simulink model "chairforceone"  (R2024a)
settings: Solver=FixedStepAuto  StartTime=0.0  StopTime=inf  RelTol=1e-3
libraries: robotlib x5
settings Model: Creator=carlosortiz  LastModifiedBy=suryachand
settings OptimizationCC: EnhancedBackFolding=on  PassReuseOutputArgsAs=Individual arguments  MaxStackSize=64  OptimizeBlockOrder=speed  DifferentSizesBufferReuse=on  OptimizationCustomize=off  EfficientTunableParamExpr=on
settings DebuggingCC: ParameterTunabilityLossMsg=error
settings HardwareCC: ProdBitPerPointer=32  ProdBitPerSizeT=32  ProdBitPerPtrDiffT=32  ProdLargestAtomicFloat=None  ProdIntDivRoundTo=Undefined  ProdEndianess=Unspecified  ProdWordSize=32  ProdHWDeviceType=Generic->Unspecified (assume 32-bit Generic)  UseEmbeddedCoderFeatures=off
settings SFSimCC: MATLABDynamicMemAlloc=off
settings RTWCC: Description=Embedded Coder  SystemTargetFile=ert.tlc  HardwareBoard=Robot Operating System (ROS)  TLCOptions="-aInlineSetEventsForThisBaseRateFcn=TLC_FALSE -aSuppressMultiTaskScheduler=TLC_FALSE  -aRateBasedStepFcn=0"  TemplateMakefile=ert_default_tmf  Toolchain=Catkin  TargetLang=C++
settings CodeAppCC: ForceParamTrailComments=on  IgnoreCustomStorageClasses=off  OperatorAnnotations=on  SimulinkDataObjDesc=on  SFDataObjDesc=on  InsertBlockDesc=on
settings ERTTargetCC: SupportNonInlinedSFcns=on

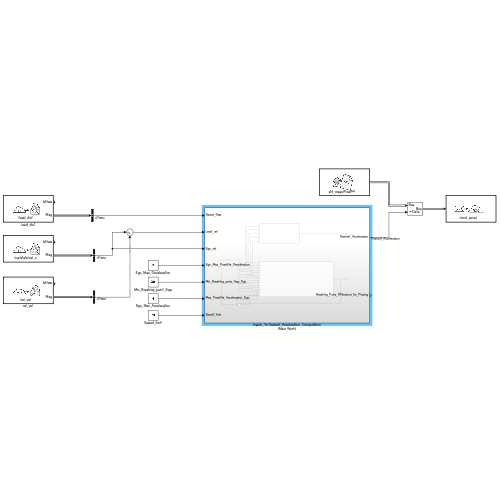
[thumbnail: Simulink's stored preview of the top-level diagram]
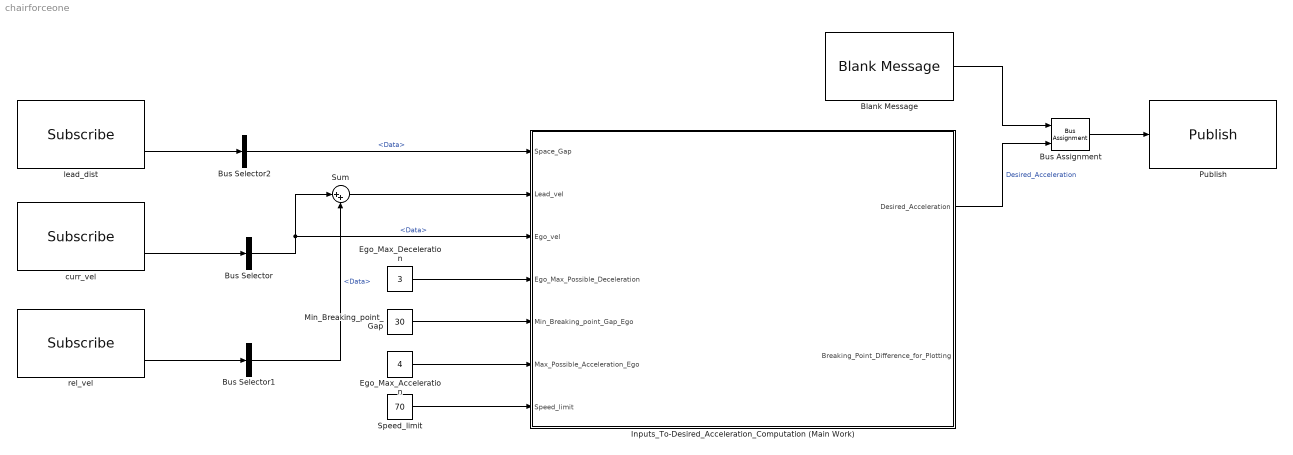
== system chairforceone ==
  Blank Message : robotlib/Blank Message  messageClass=Message  entityType=std_msgs/Float64  messageType=std_msgs/Float64  SampleTime=inf  legacyBusStruct=off
  Bus Assignment : BusAssignment  AssignedSignals=Data
  Bus Selector : BusSelector  OutputSignals=Data
  Bus Selector1 : BusSelector  OutputSignals=Data
  Bus Selector2 : BusSelector  OutputSignals=Data
  Ego_Max_Acceleration : Constant  Value=4
  Ego_Max_Deceleration : Constant  Value=3
  Inputs_To-Desired_Acceleration_Computation (Main Work) : Subsystem
  Min_Breaking_point_Gap : Constant  Value=30
  Publish : robotlib/Publish  topicSource=Specify your own  topic=/cmd_accel  messageType=std_msgs/Float64  legacyBusStruct=off  messageQueueLength=1
  Speed_limit : Constant  Value=70
  Sum : Sum  Inputs=|++
  curr_vel : robotlib/Subscribe  topicSource=Specify your own  topic=/car/state/vel_x  messageType=std_msgs/Float64  SampleTime=-1  legacyBusStruct=off  messageQueueLength=1
  lead_dist : robotlib/Subscribe  topicSource=Specify your own  topic=/lead_dist  messageType=std_msgs/Float64  SampleTime=-1  legacyBusStruct=off  messageQueueLength=1
  rel_vel : robotlib/Subscribe  topicSource=Specify your own  topic=/rel_vel  messageType=std_msgs/Float64  SampleTime=-1  legacyBusStruct=off  messageQueueLength=1
  wires:
  curr_vel/2 -> Bus Selector/1
  rel_vel/2 -> Bus Selector1/1
  lead_dist/2 -> Bus Selector2/1
  Bus Selector2/1 -> Inputs_To-Desired_Acceleration_Computation (Main Work)/1(Space_Gap)  "<Data>"
  Bus Selector/1 -> Sum/1, Inputs_To-Desired_Acceleration_Computation (Main Work)/3(Ego_vel)  "<Data>"
  Sum/1 -> Inputs_To-Desired_Acceleration_Computation (Main Work)/2(Lead_vel)
  Bus Selector1/1 -> Sum/2  "<Data>"
  Blank Message/1 -> Bus Assignment/1
  Inputs_To-Desired_Acceleration_Computation (Main Work)/1(Desired_Acceleration) -> Bus Assignment/2  "Desired_Acceleration"
  Bus Assignment/1 -> Publish/1
  Ego_Max_Deceleration/1 -> Inputs_To-Desired_Acceleration_Computation (Main Work)/4(Ego_Max_Possible_Deceleration)
  Min_Breaking_point_Gap/1 -> Inputs_To-Desired_Acceleration_Computation (Main Work)/5(Min_Breaking_point_Gap_Ego)
  Ego_Max_Acceleration/1 -> Inputs_To-Desired_Acceleration_Computation (Main Work)/6(Max_Possible_Acceleration_Ego)
  Speed_limit/1 -> Inputs_To-Desired_Acceleration_Computation (Main Work)/7(Speed_limit)

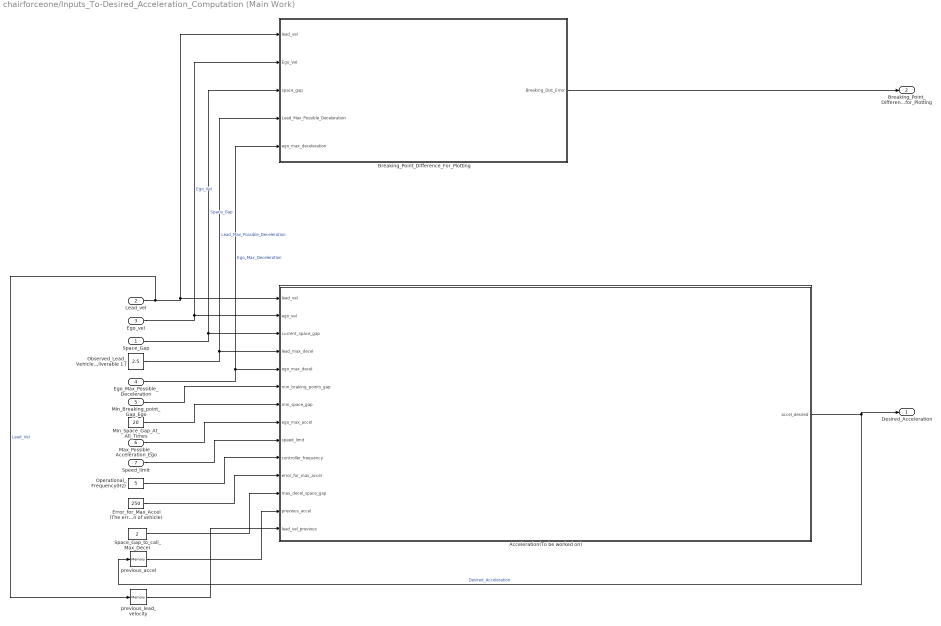
== system chairforceone/Inputs_To-Desired_Acceleration_Computation (Main Work) ==
  Space_Gap : Inport
  Lead_vel : Inport  Port=2
  Ego_vel : Inport  Port=3
  Ego_Max_Possible_Deceleration : Inport  Port=4
  Min_Breaking_point_Gap_Ego : Inport  Port=5
  Max_Possible_Acceleration_Ego : Inport  Port=6
  Speed_limit : Inport  Port=7
  Acceleration(To be worked on) : MATLAB Function  TreatAsAtomicUnit=on
  Breaking_Point_Difference_For_Plotting : Subsystem
  Error_for_Max_Accel (The error distance in breaking points which is threshold for using max acceleration of vehicle) : Constant  Value=250
  Min_Space_Gap_At_All_Times : Constant  Value=20
  Observed_Lead_Vehicle_Max_Deceleration (For now keeping one fixed value to all vehicles for scope of deliverable 1 ) : Constant  Value=2.5
  Operational_Frequency(Hz) : Constant  Value=5
  Space_Gap_to_call_Max_Decel : Constant  Value=2
  previous_accel : Memory
  previous_lead_velocity : Memory
  Desired_Acceleration : Outport
  Breaking_Point_Difference_for_Plotting : Outport  Port=2
  wires:
  Acceleration(To be worked on)/1(accel_desired) -> Desired_Acceleration/1, previous_accel/1  "Desired_Acceleration"
  Min_Breaking_point_Gap_Ego/1 -> Acceleration(To be worked on)/6(min_braking_points_gap)
  Max_Possible_Acceleration_Ego/1 -> Acceleration(To be worked on)/8(ego_max_accel)
  Speed_limit/1 -> Acceleration(To be worked on)/9(speed_limit)
  Min_Space_Gap_At_All_Times/1 -> Acceleration(To be worked on)/7(min_space_gap)
  Operational_Frequency(Hz)/1 -> Acceleration(To be worked on)/10(controller_frequency)
  Error_for_Max_Accel (The error distance in breaking points which is threshold for using max acceleration of vehicle)/1 -> Acceleration(To be worked on)/11(error_for_max_accel)
  Space_Gap_to_call_Max_Decel/1 -> Acceleration(To be worked on)/12(max_decel_space_gap)
  Space_Gap/1 -> Breaking_Point_Difference_For_Plotting/3(space_gap), Acceleration(To be worked on)/3(current_space_gap)  "Space_Gap"
  Ego_Max_Possible_Deceleration/1 -> Acceleration(To be worked on)/5(ego_max_decel), Breaking_Point_Difference_For_Plotting/5(ego_max_deceleration)  "Ego_Max_Deceleration"
  Observed_Lead_Vehicle_Max_Deceleration (For now keeping one fixed value to all vehicles for scope of deliverable 1 )/1 -> Acceleration(To be worked on)/4(lead_max_decel), Breaking_Point_Difference_For_Plotting/4(Lead_Max_Possible_Deceleration)  "Lead_Max_Possible_Deceleration"
  Ego_vel/1 -> Breaking_Point_Difference_For_Plotting/2(Ego_Vel), Acceleration(To be worked on)/2(ego_vel)  "Ego_Vel"
  Lead_vel/1 -> previous_lead_velocity/1, Breaking_Point_Difference_For_Plotting/1(lead_vel), Acceleration(To be worked on)/1(lead_vel)  "Lead_Vel"
  Breaking_Point_Difference_For_Plotting/1(Breaking_Dist_Error) -> Breaking_Point_Difference_for_Plotting/1
  previous_accel/1 -> Acceleration(To be worked on)/13(previous_accel)
  previous_lead_velocity/1 -> Acceleration(To be worked on)/14(lead_vel_previous)

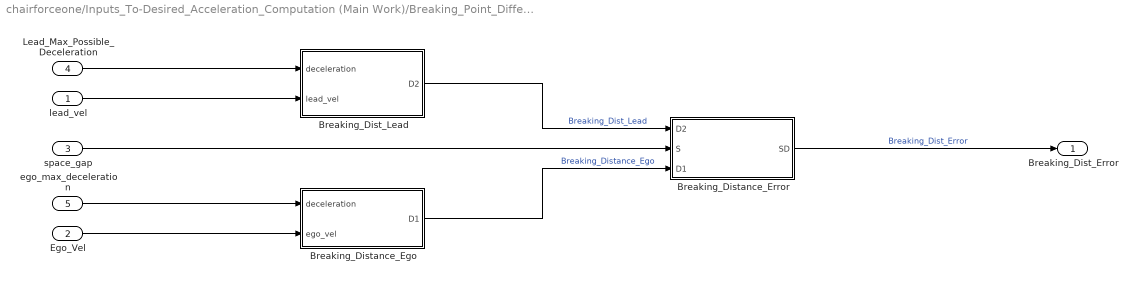
== system chairforceone/Inputs_To-Desired_Acceleration_Computation (Main Work)/Breaking_Point_Difference_For_Plotting ==
  lead_vel : Inport
  Ego_Vel : Inport  Port=2
  space_gap : Inport  Port=3
  Lead_Max_Possible_Deceleration : Inport  Port=4
  ego_max_deceleration : Inport  Port=5
  Breaking_Dist_Lead : MATLAB Function  TreatAsAtomicUnit=on
  Breaking_Distance_Ego : MATLAB Function  TreatAsAtomicUnit=on
  Breaking_Distance_Error : MATLAB Function  TreatAsAtomicUnit=on
  Breaking_Dist_Error : Outport
  wires:
  Ego_Vel/1 -> Breaking_Distance_Ego/2(ego_vel)
  space_gap/1 -> Breaking_Distance_Error/2(S)
  lead_vel/1 -> Breaking_Dist_Lead/2(lead_vel)
  ego_max_deceleration/1 -> Breaking_Distance_Ego/1(deceleration)
  Breaking_Distance_Error/1(SD) -> Breaking_Dist_Error/1  "Breaking_Dist_Error"
  Breaking_Distance_Ego/1(D1) -> Breaking_Distance_Error/3(D1)  "Breaking_Distance_Ego"
  Lead_Max_Possible_Deceleration/1 -> Breaking_Dist_Lead/1(deceleration)
  Breaking_Dist_Lead/1(D2) -> Breaking_Distance_Error/1(D2)  "Breaking_Dist_Lead"

== matlab function chairforceone/Inputs_To-Desired_Acceleration_Computation (Main Work)/Acceleration(To be worked on) ==
  data: accel_desired output; lead_vel input; ego_vel input; current_space_gap input; lead_max_decel input; ego_max_decel input; min_braking_points_gap input; min_space_gap input; ego_max_accel input; speed_limit input; controller_frequency input; error_for_max_accel input; max_decel_space_gap input; previous_accel input; lead_vel_previous input
function accel_desired = accel_ctrl_(lead_vel, ego_vel, current_space_gap, ...
    lead_max_decel, ego_max_decel, min_braking_points_gap, min_space_gap, ...
    ego_max_accel, speed_limit, controller_frequency, error_for_max_accel, max_decel_space_gap, previous_accel, lead_vel_previous)
    % ACCEL_CTRL_ Calculates the desired acceleration for the ego vehicle to maintain
    % a safe following distance behind a lead vehicle while considering vehicle capabilities
    % and safety constraints.
    %
    % Parameters:
    %   lead_vel                - Velocity of the lead vehicle (m/s)
    %   ego_vel                 - Current velocity of the ego vehicle (m/s)
    %   current_space_gap       - Current distance between ego and lead vehicles (m)
    %   lead_max_decel          - Maximum deceleration capability of the lead vehicle (m/s²)
    %   ego_max_decel           - Maximum deceleration capability of the ego vehicle (m/s²)
    %   min_braking_points_gap  - Minimum desired gap based on braking points (m)
    %   min_space_gap           - Absolute minimum safe space gap (m)
    %   ego_max_accel           - Maximum acceleration capability of the ego vehicle (m/s²)
    %   speed_limit             - Speed limit of the road (m/s) [Not used in current implementation]
    %   controller_frequency    - Frequency at which the controller operates (Hz)
    %   error_for_max_accel     - Error threshold at which maximum acceleration is applied (m)
    %   max_decel_space_gap     - Additional space gap for maximum deceleration (m)
    %
    % Returns:
    %   accel_desired - The desired acceleration command for the ego vehicle (m/s²)
    
    % Constants
    epsilon = 1e-3; % Small value for floating-point comparison
    f = 0.55; % Coefficient of friction between tires and road
    g = 9.8;  % Acceleration due to gravity (m/s²)

    % Time step calculation based on controller frequency
    dt = 1 / controller_frequency;

    % Step 0: Handle No Lead Vehicle Case
    % -----------------------------------
    relvel = ego_vel - lead_vel;
    if (abs(relvel) < epsilon) && (current_space_gap > 250)
        % No significant lead vehicle influence
        % Accelerate towards speed limit or maintain it if already reached
        if ego_vel < speed_limit
            % Calculate the required acceleration to reach speed limit smoothly
            accel_desired = min(ego_max_accel, (speed_limit - ego_vel) / dt);
        else
            % Maintain speed limit
            accel_desired = 0;
        end

        % Ensure accel_desired does not exceed vehicle's capabilities
        accel_desired = min(accel_desired, ego_max_accel);
        accel_desired = max(accel_desired, -ego_max_decel);

        % Apply Low-Pass Filter to Smooth Acceleration Changes Only if Signs Match
        % -----------------------------------------------------------------------
        % Determine the signs of current and previous acceleration
        sign_accel_desired = sign(accel_desired);
        sign_previous_accel = sign(previous_accel);
        
        % If the acceleration sign changes, reset previous_accel to zero
        if sign_accel_desired * sign_previous_accel < 0 % Signs are different
            previous_accel = 0;
        end
        
        % Apply Low-Pass Filter to Smooth Acceleration Changes
        alpha = 0.3; % Adjusted smoothing factor for acceleration
        accel_desired = alpha * accel_desired + (1 - alpha) * previous_accel;

        return;
    end

    % Step 1: Initialize Working Variables
    % -------------------------------------
    % These variables may be adjusted based on the relative deceleration capabilities
    % of the ego and lead vehicles.
    working_decel_ego = ego_max_decel;   % Working maximum deceleration of ego vehicle
    working_decel_lead = lead_max_decel; % Working maximum deceleration of lead vehicle
    working_min_gap = min_braking_points_gap; % Minimum braking point gap

    % Conditional Adjustment Based on Maximum Decelerations
    if ego_max_decel > lead_max_decel
        % If ego vehicle can decelerate faster than lead vehicle,
        % limit ego's deceleration to lead's maximum deceleration to maintain safety.
        working_decel_ego = lead_max_decel;

        % Adjust the working minimum gap to ensure safety
        working_min_gap = min(min_space_gap, min_braking_points_gap);
    end

    % Step 2: Calculate Stopping Distances
    % -------------------------------------
    % Calculate the stopping distances for both ego and lead vehicles.
    D1 = (ego_vel^2 / (2 * working_decel_ego)) + ((ego_vel^2 / (2 * g)) * f);
    D2 = (lead_vel^2 / (2 * working_decel_lead)) + ((lead_vel^2 / (2 * g)) * f);

    % Step 3: Compute the Stopping Distance Error
    % -------------------------------------------
    % Determine how much the current stopping distance deviates from the desired minimum gap.
    stop_dist = (D2 + current_space_gap) - D1;
    error = stop_dist - working_min_gap;

    % Step 4: Map Error to Desired Acceleration Using Different Gamma Values
    % ------------------------------------------------------------------------
    % Adjusted Parameters for Balanced Responsiveness
    gamma_neg = 0.5; % Increased from 0.1 for softer deceleration
    gamma_pos = 1.1; % Reduced from 1.5 for balanced acceleration

    threshold_decel_error = -(working_min_gap - max_decel_space_gap); % Negative threshold
    threshold_accel_error = error_for_max_accel; % Positive threshold

    if error >= threshold_accel_error
        % Case 1: Error exceeds the positive threshold
        % Apply maximum acceleration.
        accel_desired = ego_max_accel;
    elseif error >= 0
        % Case 2: Error is positive but below the threshold
        % Apply a non-linear (linear in this case) mapping to determine desired acceleration.
        accel_desired = ego_max_accel * (error / threshold_accel_error)^gamma_pos;
    elseif error <= threshold_decel_error
        % Case 3: Error exceeds the negative threshold
        % Apply maximum deceleration.
        accel_desired = -ego_max_decel;
    else
        % Case 4: Error is negative but above the threshold
        % Apply a non-linear (softer) mapping to determine desired deceleration.
        accel_desired = -ego_max_decel * (error / threshold_decel_error)^gamma_neg;
    end

    % New Step: Apply Low-Pass Filter to Smooth Acceleration Changes
    % --------------------------------------------------------------
    % Enhanced Smoothing with Dynamic Factors
    if accel_desired > -ego_max_decel
        % Determine the signs of current and previous acceleration
        sign_accel_desired = sign(accel_desired);
        sign_previous_accel = sign(previous_accel);
        
        % If the acceleration sign changes, reset previous_accel to zero
        if sign_accel_desired * sign_previous_accel < 0 % Signs are different
            previous_accel = 0;
        end
        
        % Apply different smoothing factors for acceleration and deceleration
        if accel_desired >= 0
            alpha = 0.3; % Smoothing factor for acceleration
        else
            alpha = 0.6; % Smoothing factor for deceleration
        end
        
        % Apply Low-Pass Filter
        accel_desired = alpha * accel_desired + (1 - alpha) * previous_accel;
    end

    % Step 5: Weighted Multiple Time Step Lookahead
    % ---------------------------------------------
    
    % Define the number of steps to look ahead
    n_steps = 1; % Number of lookahead steps (adjustable)
    dt = 1 / controller_frequency; % Time step
    
    % Define weights for each future time step
    lambda = 0.8; % Decay rate (adjustable)
    weights = lambda .^ (0:n_steps-1);
    weights = weights / sum(weights); % Normalize weights to sum to 1
    
    % Compute lead acceleration
    lead_accel = (lead_vel - lead_vel_previous) / dt;
    
    % Initialize variables for future positions and velocities
    ego_future_pos = 0; % Assuming current position is 0
    lead_future_pos = current_space_gap; % Starting from current space gap
    ego_future_vel = ego_vel;
    lead_future_vel = lead_vel;
    
    % Initialize an array to store future space gaps
    future_space_gaps = zeros(1, n_steps);
    
    % Simulate over n_steps to predict future positions
    for i = 1:n_steps
        % Predict future acceleration for ego vehicle
        % For prediction, assume current accel_desired remains constant
        ego_future_vel = ego_future_vel + accel_desired * dt;
        ego_future_pos = ego_future_pos + ego_future_vel * dt + 0.5 * accel_desired * dt^2;
        
        % Predict future acceleration for lead vehicle
        % Assume constant lead_accel
        lead_future_vel = lead_future_vel + lead_accel * dt;
        lead_future_pos = lead_future_pos + lead_future_vel * dt + 0.5 * lead_accel * dt^2;
        
        % Compute future space gap at this time step
        future_space_gaps(i) = lead_future_pos - ego_future_pos;
    end
    
    % Apply weights to future space gaps
    weighted_future_gap = sum(weights .* future_space_gaps);
    
    % Initialize flag to track if accel_desired is updated in lookahead
    accel_updated_in_lookahead = false;

    % Step 6: Adjust Desired Acceleration Based on Weighted Future Gap
    % ---------------------------------------------------------------
    
    if weighted_future_gap < min_space_gap
        % Calculate the required deceleration to maintain the minimum space gap
        required_distance = weighted_future_gap - min_space_gap;
        relative_velocity = ego_future_vel - lead_future_vel;

        % Compute the required deceleration using kinematic equations
        if required_distance < 0
            % Need to decelerate more to avoid collision
            decel_required = (relative_velocity^2) / (2 * abs(required_distance));
            accel_required = -decel_required; % Deceleration is negative acceleration

            % Update accel_desired if more deceleration is needed
            if accel_required < accel_desired
                accel_desired = accel_required;
                % Set flag to indicate that accel_desired was updated
                accel_updated_in_lookahead = true;
            end
        end
    end

    % Step 7: Apply Smoothing to Acceleration Commands Conditionally
    % -------------------------------------------------------------
    
    if accel_updated_in_lookahead
        smoothing_factor = 0.4; % Smoothing factor between 0 and 1 (adjustable)
        accel_desired = smoothing_factor * accel_desired + (1 - smoothing_factor) * previous_accel;
    end

    % Step 8: Prevent Deceleration When Velocity Is Zero
    % -------------------------------------------------
    
    velocity_epsilon = 1e-3; % Threshold to consider vehicle at rest
    if ego_vel <= velocity_epsilon && accel_desired < 0
        % Vehicle is at rest; do not command further deceleration
        accel_desired = 0;
    end

    % Step 9: Final Clipping of Desired Acceleration with Rate Limiting
    % --------------------------------------------------------------
    
    % Implement Rate Limiting
    max_accel_change = 1.0; % m/s² per controller step (adjustable)
    desired_change = accel_desired - previous_accel;
    
    if desired_change > max_accel_change
        accel_desired = previous_accel + max_accel_change;
    elseif desired_change < -max_accel_change
        accel_desired = previous_accel - max_accel_change;
    end
    
    % Final Clipping to Ensure Within Vehicle's Capabilities
    accel_desired = min(accel_desired, ego_max_accel);    % Limit to maximum acceleration
    accel_desired = max(accel_desired, -ego_max_decel);   % Limit to maximum deceleration
end

== matlab function chairforceone/Inputs_To-Desired_Acceleration_Computation (Main Work)/Breaking_Point_Difference_For_Plotting/Breaking_Distance_Error ==
  data: D2 input; SD output; S input; D1 input
function SD = stop_dist_diff(D2, S, D1)

SD = (D2+S)-D1;

== matlab function chairforceone/Inputs_To-Desired_Acceleration_Computation (Main Work)/Breaking_Point_Difference_For_Plotting/Breaking_Distance_Ego ==
  data: deceleration input; D1 output; ego_vel input
function D1 = D1(deceleration, ego_vel)
    f=0.55; % coeff. friction
    g=9.8;
    D1 = (ego_vel^2 / (2*deceleration))+((ego_vel^2/(2*g))*f);

== matlab function chairforceone/Inputs_To-Desired_Acceleration_Computation (Main Work)/Breaking_Point_Difference_For_Plotting/Breaking_Dist_Lead ==
  data: deceleration input; lead_vel input; D2 output
function D2 = D2(deceleration, lead_vel)
    f=0.55; % coeff. friction
    g=9.8;
    D2 = (lead_vel^2 / (2*deceleration))+((lead_vel^2/(2*g))*f);
